simulink model "Full"  (R2014b)
settings: Solver=ode45  StartTime=5  StopTime=Timemax  RelTol=1e-3
values from neighbouring files (symbols this model uses):
  params = fillPosEstimatorInavParams(Par)    [a_log_read.m]
  SampleTime = ts    [a_log_read.m]
undefined symbols (not defined in the file or in its folder): Par, ts
libraries: mylib x10, dspsigattribs x1
settings Model: Creator=Marat  LastModifiedBy=Marat

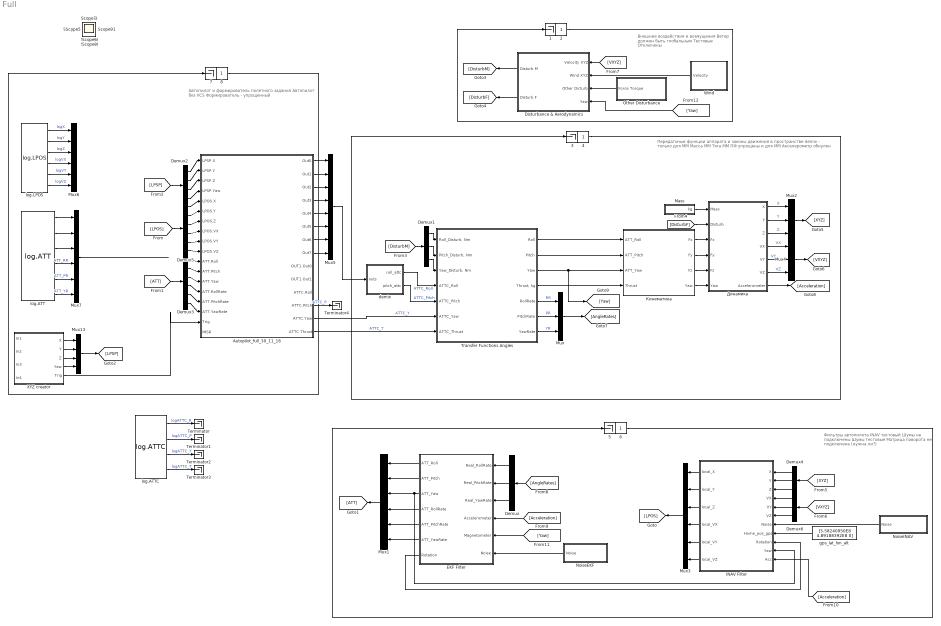
== system Full ==
  note: Передатоные функции аппарата и законы движения в пространстве
      | demix - только для ММ
      | Масса ММ
      | Тяга ММ
      | ПФ упрощены и для ММ
      | Акселерометр обнулен
  note: Внешние воздействия и возмущения
      | Ветер должен быть глобальным
      | Тестовые
      | Отключены
  note: Фильтры автопилота
      | INAV тестовый
      | Шумы не подключены
      | Шумы тестовые
      | Матрица поворота не подключена (нужна ли?)
  note: Автопилот и формирователь полетного задания
      | Автопилот без VCS
      | Формирователь - упрощенный
  {1,3,5,7} (4 alike) : Terminator
  {2,4,6,8} (4 alike) : Constant
  Autopilot_full_30_11_16 : Subsystem  AncestorBlock=mylib/Autopilot_full_30_11_16  mask(Автопилот полный pos + attitude){}
      mask help:
      | Автопилот полный 30.11.16 для анализа в полном автомате
      | (полет по GPS)
      mask Help:
      | Автор - М.Сабиров
      | 30.11.16
  Demux{,1,4,6} (4 alike) : Demux  Outputs=3
  Demux2 : Demux
  Demux3 : Demux  Outputs=6
  Demux5 : Demux  Outputs=6
  Disturbance & Aerodynamics : Subsystem
  EKF Filter : Subsystem
  INAV Filter : Subsystem
  Mass : Subsystem
  Mux : Mux  Inputs=3
  Mux{1,3,6..7} (4 alike) : Mux  Inputs=6
  Mux13 : Mux
  Mux2 : Mux  Inputs=3
  Mux4 : Mux  Inputs=3
  Mux5 : Mux  Inputs=8
  NoiseEKF : Subsystem
  NoiseINAV : Subsystem
  Other Disturbance : Subsystem
  Terminator{,1..4} (5 alike) : Terminator
  Transfer Functions Angles : Subsystem
  Wind : Subsystem
  XYZ creator : Subsystem
  demix : Subsystem
  gps_lat_lon_alt : Constant  Value=[5.58240950E8 4.89188392E8 0]
  log.ATT : mylib/Log_read/log.ATT
  log.ATTC : mylib/Log_read/log.ATTC
  log.LPOS : mylib/Log_read/log.LPOS
  Динамика : Subsystem
  Кинематика : MATLAB Function  TreatAsAtomicUnit=on
  Scope{,1..13} (14 alike) : Scope
      Scope settings: ShowLegends=on  YMin=-2.5  YMax=2.5
      Scope1 settings: ShowLegends=on  YMin=-2  YMax=1
      Scope10 settings: ShowLegends=on  YMin=-0.5  YMax=0.4  SaveName=ScopeData14
      Scope11 settings: ShowLegends=on  YMin=-0.3  YMax=0.4  SaveName=ScopeData17
      Scope12 settings: ShowLegends=on  YMin=-6  YMax=8  SaveName=ScopeData19
      Scope13 settings: ShowLegends=on  SaveName=ScopeData20
      Scope2 settings: ShowLegends=on  YMin=-0.5  YMax=0.2  SaveName=ScopeData2
      Scope3 settings: SaveName=ScopeData3
      Scope4 settings: ShowLegends=on  YMin=-2.5  YMax=0.5  SaveName=ScopeData4
      Scope5 settings: ShowLegends=on  YMin=0.65  YMax=0.95  SaveName=ScopeData6
      Scope6 settings: ShowLegends=on  SaveName=ScopeData18
      Scope7 settings: ShowLegends=on  YMin=-12  YMax=0  SaveName=ScopeData8
      Scope8 settings: ShowLegends=on  TimeRange=19.50883891213388  YMin=-0.18  YMax=-0.04  SaveName=ScopeData11
      Scope9 settings: ShowLegends=on  TimeRange=102.475  YMin=-30  YMax=15  SaveName=ScopeData12
  wires:
  Autopilot_full_30_11_16/13(ATTC.Yaw) -> Transfer Functions Angles/6(ATTC_Yaw)  "ATTC_Y"
  Autopilot_full_30_11_16/14(ATTC.Thrust) -> Transfer Functions Angles/7(ATTC_Thrust)  "ATTC_T"
  Transfer Functions Angles/7(YawRate) -> Mux/3  "YR"
  Transfer Functions Angles/6(PitchRate) -> Mux/2  "PR"
  Transfer Functions Angles/5(RollRate) -> Mux/1  "RR"
  Demux/1 -> EKF Filter/1(Real_RollRate)
  Demux/2 -> EKF Filter/2(Real_PitchRate)
  Demux/3 -> EKF Filter/3(Real_YawRate)
  Demux1/3 -> Transfer Functions Angles/3("Yaw_Disturb, Nm")
  Demux1/2 -> Transfer Functions Angles/2("Pitch_Disturb, Nm")
  Demux1/1 -> Transfer Functions Angles/1("Roll_Disturb, Nm")
  EKF Filter/1(ATT_Roll) -> Mux1/1
  EKF Filter/6(ATT_YawRate) -> Mux1/6
  Demux3/1 -> Autopilot_full_30_11_16/11(ATT.Roll)
  Demux3/6 -> Autopilot_full_30_11_16/16(ATT.YawRate)
  Demux3/5 -> Autopilot_full_30_11_16/15(ATT.PitchRate)
  Demux3/4 -> Autopilot_full_30_11_16/14(ATT.RollRate)
  Demux3/3 -> Autopilot_full_30_11_16/13(ATT.Yaw)
  Demux3/2 -> Autopilot_full_30_11_16/12(ATT.Pitch)
  EKF Filter/2(ATT_Pitch) -> Mux1/2
  EKF Filter/3(ATT_Yaw) -> INAV Filter/10(Yaw), Mux1/3
  EKF Filter/4(ATT_RollRate) -> Mux1/4
  EKF Filter/5(ATT_PitchRate) -> Mux1/5
  Transfer Functions Angles/1(Roll) -> Кинематика/1(ATT_Roll)
  Transfer Functions Angles/2(Pitch) -> Кинематика/2(ATT_Pitch)
  Transfer Functions Angles/3(Yaw) -> Кинематика/3(ATT_Yaw), [Yaw]
  Кинематика/1(Fx) -> Динамика/3(Fx)
  Кинематика/2(Fy) -> Динамика/4(Fy)
  Динамика/1(X) -> Mux2/1  "X"
  Динамика/2(Y) -> Mux2/2  "Y"
  Динамика/3(Z) -> Mux2/3  "Z"
  Динамика/4(VX) -> Mux4/1  "VX"
  Динамика/5(VY) -> Mux4/2  "VY"
  Динамика/6(VZ) -> Mux4/3  "VZ"
  Demux4/1 -> INAV Filter/1(X)
  Demux6/3 -> INAV Filter/6(VZ)
  Demux6/2 -> INAV Filter/5(VY)
  Demux6/1 -> INAV Filter/4(VX)
  Demux4/3 -> INAV Filter/3(Z)
  INAV Filter/1(local_X) -> Mux3/1
  INAV Filter/6(local_VZ) -> Mux3/6
  INAV Filter/2(local_Y) -> Mux3/2
  INAV Filter/3(local_Z) -> Mux3/3
  INAV Filter/4(local_VX) -> Mux3/4
  INAV Filter/5(local_VY) -> Mux3/5
  Demux4/2 -> INAV Filter/2(Y)
  Demux5/1 -> Autopilot_full_30_11_16/5(LPOS.X)
  Demux5/6 -> Autopilot_full_30_11_16/10(LPOS.VZ)
  Demux5/5 -> Autopilot_full_30_11_16/9(LPOS.VY)
  Demux5/4 -> Autopilot_full_30_11_16/8(LPOS.VX)
  Demux5/3 -> Autopilot_full_30_11_16/7(LPOS.Z)
  Demux5/2 -> Autopilot_full_30_11_16/6(LPOS.Y)
  Other Disturbance/1(Force Torque) -> Disturbance & Aerodynamics/3(Other Dicturb)
  NoiseINAV/1(Noise) -> INAV Filter/7(Noise)
  NoiseEKF/1(Noise) -> EKF Filter/6(Noise)
  EKF Filter/7(Rotation) -> INAV Filter/9(Rotation)
  gps_lat_lon_alt/1 -> INAV Filter/8(Home_pos_gps)
  XYZ creator/5(Trig) -> Autopilot_full_30_11_16/17(Trig)
  log.LPOS/1 -> Mux6/1  "logX"
  log.LPOS/6 -> Mux6/6  "logVZ"
  log.LPOS/2 -> Mux6/2  "logY"
  log.LPOS/3 -> Mux6/3  "logZ"
  log.LPOS/4 -> Mux6/4  "logVX"
  log.LPOS/5 -> Mux6/5  "logVY"
  log.ATT/1 -> Mux7/1
  log.ATT/2 -> Mux7/2
  log.ATT/3 -> Mux7/3
  log.ATT/4 -> Mux7/4  "ATT_RR"
  log.ATT/5 -> Mux7/5  "ATT_PR"
  log.ATT/6 -> Mux7/6  "ATT_YR"
  [LPOS] -> Demux5/1
  Mux3/1 -> [LPOS]
  Mux7/1 -> ?
  Mux1/1 -> [ATT]
  XYZ creator/1(X) -> Mux13/1
  XYZ creator/2(Y) -> Mux13/2
  XYZ creator/3(Z) -> Mux13/3
  XYZ creator/4(Yaw) -> Mux13/4
  Demux2/4 -> Autopilot_full_30_11_16/4(LPSP.Yaw)
  Demux2/1 -> Autopilot_full_30_11_16/1(LPSP.X)
  Demux2/2 -> Autopilot_full_30_11_16/2(LPSP.Y)
  Demux2/3 -> Autopilot_full_30_11_16/3(LPSP.Z)
  Mux13/1 -> [LPSP]
  [LPSP] -> Demux2/1
  [DisturbM] -> Demux1/1
  Disturbance & Aerodynamics/1(Disturb M) -> [DisturbM]
  Disturbance & Aerodynamics/2(Disturb F) -> [DisturbF]
  [DisturbF] -> Динамика/2(Disturb)
  Mux2/1 -> [XYZ]
  [XYZ] -> Demux4/1
  Mux4/1 -> [VXYZ]
  [VXYZ] -> Demux6/1
  [VXYZ] -> Disturbance & Aerodynamics/1(Velocity XYZ)
  Mux/1 -> [AngleRates]
  [AngleRates] -> Demux/1
  Динамика/7(Accelerometer) -> [Acceleration]
  [Acceleration] -> EKF Filter/4(Accelerometer)
  [Acceleration] -> INAV Filter/11(Acc)
  [Yaw] -> EKF Filter/5(Magnetometer)
  4/1 -> 3/1
  6/1 -> 5/1
  2/1 -> 1/1
  8/1 -> 7/1
  log.ATTC/1 -> Terminator/1  "logATTC_R"
  log.ATTC/2 -> Terminator1/1  "logATTC_P"
  log.ATTC/3 -> Terminator2/1  "logATTC_Y"
  log.ATTC/4 -> Terminator3/1  "logATTC_T"
  demix/2(pitch_attc) -> Transfer Functions Angles/5(ATTC_Pitch)  "ATTC_Pitch"
  Autopilot_full_30_11_16/1(Out0) -> Mux5/1
  Autopilot_full_30_11_16/8(Out7) -> Mux5/8
  Autopilot_full_30_11_16/2(Out1) -> Mux5/2
  Autopilot_full_30_11_16/3(Out2) -> Mux5/3
  Autopilot_full_30_11_16/5(Out4) -> Mux5/5
  Autopilot_full_30_11_16/7(Out6) -> Mux5/7
  Autopilot_full_30_11_16/6(Out5) -> Mux5/6
  Autopilot_full_30_11_16/4(Out3) -> Mux5/4
  Mux5/1 -> demix/1(outs)
  demix/1(roll_attc) -> Transfer Functions Angles/4(ATTC_Roll)  "ATTC_Roll"
  Mass/1(kg) -> Динамика/1(Mass)
  [Yaw] -> Disturbance & Aerodynamics/4(Yaw)
  Wind/1(Velocity) -> Disturbance & Aerodynamics/2(Wind XYZ)
  Autopilot_full_30_11_16/12(ATTC.Pitch) -> Terminator4/1  "ATTC_P"
  [ATT] -> Demux3/1
  Transfer Functions Angles/4("Thrust, kg") -> Кинематика/4(Thrust)
  Кинематика/3(Fz) -> Динамика/5(Fz)
  Кинематика/4(Yaw) -> Динамика/6(Yaw)

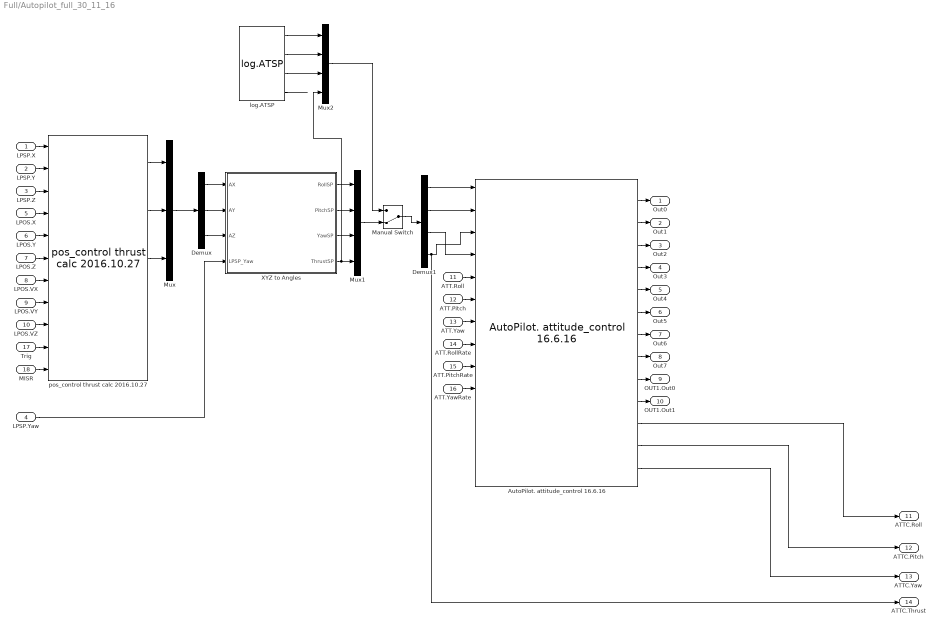
== system Full/Autopilot_full_30_11_16 ==
  LPSP.X : Inport
  LPSP.Y : Inport  Port=2
  LPSP.Z : Inport  Port=3
  LPSP.Yaw : Inport  Port=4
  LPOS.X : Inport  Port=5
  LPOS.Y : Inport  Port=6
  LPOS.Z : Inport  Port=7
  LPOS.VX : Inport  Port=8
  LPOS.VY : Inport  Port=9
  LPOS.VZ : Inport  Port=10
  ATT.Roll : Inport  Port=11
  ATT.Pitch : Inport  Port=12
  ATT.Yaw : Inport  Port=13
  ATT.RollRate : Inport  Port=14
  ATT.PitchRate : Inport  Port=15
  ATT.YawRate : Inport  Port=16
  Trig : Inport  Port=17
  MISR : Inport  Port=18
  AutoPilot. attitude_control 16.6.16 : mylib/AutoPilot. attitude_control  16.6.16  log_model=off  mm_model=off  rotation_yaw=on
  Demux : Demux  Outputs=3
  Demux1 : Demux
  Manual Switch : ManualSwitch  CurrentSetting=0
  Mux : Mux  Inputs=3
  Mux1 : Mux
  Mux2 : Mux
  XYZ to Angles : MATLAB Function  TreatAsAtomicUnit=on  mask(Преобразование желаемого вектора тяги в углы управления){}
      mask help:
      | Входами блока являются выходы Pos_Control:
      |     AX - проекция желаемой тяги на Х
      |     AY - проекция желаемой тяги на Y
      |     AZ - проекция желаемой тяги на Z
      | и желаемое рыскание LPSP.Yaw
      |
      | Выходами блока являются входы Att_Control:
      |     RollSP - желаемый угол наклона по крену,
      |     PitchSP - желаемый угол наклона по тангажу,
      |     YawSP  - желаемый угол наклона по рысканию,
      |     ThrustSP - желаемая тяга.
  log.ATSP : mylib/Log_read/log.ATSP
  pos_control thrust calc 2016.10.27 : mylib/pos_control thrust calc 2016.10.27
  Out0 : Outport
  Out1 : Outport  Port=2
  Out2 : Outport  Port=3
  Out3 : Outport  Port=4
  Out4 : Outport  Port=5
  Out5 : Outport  Port=6
  Out6 : Outport  Port=7
  Out7 : Outport  Port=8
  OUT1.Out0 : Outport  Port=9
  OUT1.Out1 : Outport  Port=10
  ATTC.Roll : Outport  Port=11
  ATTC.Pitch : Outport  Port=12
  ATTC.Yaw : Outport  Port=13
  ATTC.Thrust : Outport  Port=14
  wires:
  AutoPilot. attitude_control 16.6.16/10 -> OUT1.Out1/1
  AutoPilot. attitude_control 16.6.16/9 -> OUT1.Out0/1
  pos_control thrust calc 2016.10.27/1 -> Mux/1
  pos_control thrust calc 2016.10.27/2 -> Mux/2
  pos_control thrust calc 2016.10.27/3 -> Mux/3
  Mux/1 -> Demux/1
  Demux/1 -> XYZ to Angles/1(AX)
  Demux/2 -> XYZ to Angles/2(AY)
  Demux/3 -> XYZ to Angles/3(AZ)
  XYZ to Angles/1(RollSP) -> Mux1/1
  XYZ to Angles/2(PitchSP) -> Mux1/2
  XYZ to Angles/3(YawSP) -> Mux1/3
  XYZ to Angles/4(ThrustSP) -> Mux2/4, Mux1/4
  Demux1/1 -> AutoPilot. attitude_control 16.6.16/1
  Demux1/2 -> AutoPilot. attitude_control 16.6.16/2
  Demux1/3 -> AutoPilot. attitude_control 16.6.16/4
  Demux1/4 -> ATTC.Thrust/1, AutoPilot. attitude_control 16.6.16/3
  Mux1/1 -> Manual Switch/2
  ATT.Pitch/1 -> AutoPilot. attitude_control 16.6.16/6
  ATT.YawRate/1 -> AutoPilot. attitude_control 16.6.16/10
  ATT.PitchRate/1 -> AutoPilot. attitude_control 16.6.16/9
  ATT.Yaw/1 -> AutoPilot. attitude_control 16.6.16/7
  ATT.RollRate/1 -> AutoPilot. attitude_control 16.6.16/8
  ATT.Roll/1 -> AutoPilot. attitude_control 16.6.16/5
  LPOS.VX/1 -> pos_control thrust calc 2016.10.27/7
  AutoPilot. attitude_control 16.6.16/11 -> ATTC.Roll/1
  LPOS.VZ/1 -> pos_control thrust calc 2016.10.27/9
  AutoPilot. attitude_control 16.6.16/1 -> Out0/1
  LPOS.VY/1 -> pos_control thrust calc 2016.10.27/8
  LPOS.Y/1 -> pos_control thrust calc 2016.10.27/5
  LPOS.X/1 -> pos_control thrust calc 2016.10.27/4
  LPOS.Z/1 -> pos_control thrust calc 2016.10.27/6
  AutoPilot. attitude_control 16.6.16/5 -> Out4/1
  AutoPilot. attitude_control 16.6.16/8 -> Out7/1
  AutoPilot. attitude_control 16.6.16/6 -> Out5/1
  AutoPilot. attitude_control 16.6.16/3 -> Out2/1
  AutoPilot. attitude_control 16.6.16/2 -> Out1/1
  AutoPilot. attitude_control 16.6.16/7 -> Out6/1
  AutoPilot. attitude_control 16.6.16/4 -> Out3/1
  AutoPilot. attitude_control 16.6.16/12 -> ATTC.Pitch/1
  AutoPilot. attitude_control 16.6.16/13 -> ATTC.Yaw/1
  LPSP.Yaw/1 -> XYZ to Angles/4(LPSP_Yaw)
  LPSP.Y/1 -> pos_control thrust calc 2016.10.27/2
  LPSP.Z/1 -> pos_control thrust calc 2016.10.27/3
  LPSP.X/1 -> pos_control thrust calc 2016.10.27/1
  Trig/1 -> pos_control thrust calc 2016.10.27/10
  MISR/1 -> pos_control thrust calc 2016.10.27/11
  log.ATSP/1 -> Mux2/1
  log.ATSP/2 -> Mux2/2
  log.ATSP/3 -> Mux2/3
  log.ATSP/4 -> ?
  Mux2/1 -> Manual Switch/1
  Manual Switch/1 -> Demux1/1

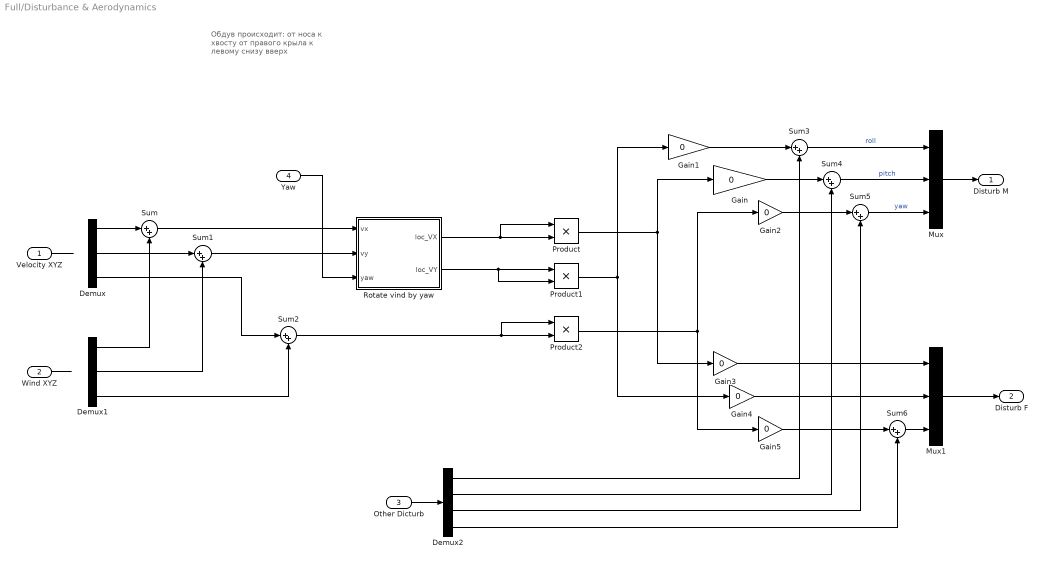
== system Full/Disturbance & Aerodynamics ==
  note: Обдув происходит:
      | от носа к хвосту
      | от правого крыла к левому
      | снизу вверх
  Velocity XYZ : Inport
  Wind XYZ : Inport  Port=2
  Other Dicturb : Inport  Port=3
  Yaw : Inport  Port=4
  Demux : Demux  Outputs=3
  Demux1 : Demux  Outputs=3
  Demux2 : Demux
  Gain{,1..5} (6 alike) : Gain  Gain=0
  Mux : Mux  Inputs=3
  Mux1 : Mux  Inputs=3
  Product : Product
  Product1 : Product
  Product2 : Product
  Rotate vind by yaw : MATLAB Function  TreatAsAtomicUnit=on
  Sum{,1..6} (7 alike) : Sum  Inputs=|++
  Disturb M : Outport
  Disturb F : Outport  Port=2
  wires:
  Mux/1 -> Disturb M/1
  Mux1/1 -> Disturb F/1
  Velocity XYZ/1 -> ?
  Wind XYZ/1 -> ?
  Demux/1 -> Sum/1
  Demux1/1 -> Sum/2
  Demux/2 -> Sum1/1
  Demux1/2 -> Sum1/2
  Demux/3 -> Sum2/1
  Demux1/3 -> Sum2/2
  Sum/1 -> Rotate vind by yaw/1(vx)
  Sum1/1 -> Rotate vind by yaw/2(vy)
  Yaw/1 -> Rotate vind by yaw/3(yaw)
  Rotate vind by yaw/1(loc_VX) -> Product/1, Product/2
  Rotate vind by yaw/2(loc_VY) -> Product1/2, Product1/1
  Sum2/1 -> Product2/1, Product2/2
  Product/1 -> Gain3/1, Gain/1
  Product1/1 -> Gain4/1, Gain1/1
  Product2/1 -> Gain5/1, Gain2/1
  Sum4/1 -> Mux/2  "pitch"
  Sum3/1 -> Mux/1  "roll"
  Sum5/1 -> Mux/3  "yaw"
  Gain3/1 -> Mux1/1
  Gain4/1 -> Mux1/2
  Gain5/1 -> Sum6/1
  Gain2/1 -> Sum5/1
  Gain/1 -> Sum4/1
  Gain1/1 -> Sum3/1
  Other Dicturb/1 -> Demux2/1
  Demux2/1 -> Sum3/2
  Demux2/2 -> Sum4/2
  Demux2/3 -> Sum5/2
  Sum6/1 -> Mux1/3
  Demux2/4 -> Sum6/2

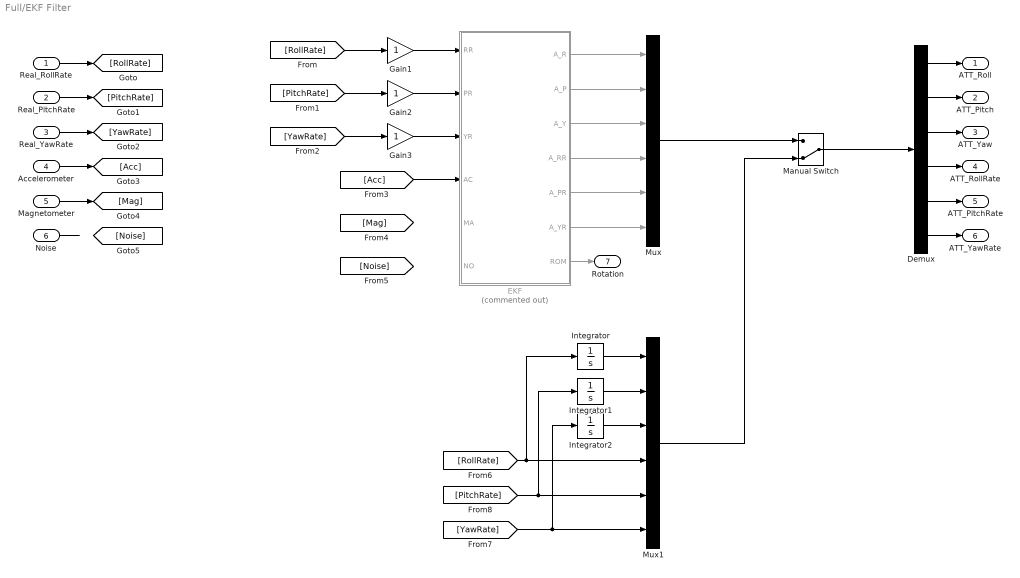
== system Full/EKF Filter ==
  Real_RollRate : Inport
  Real_PitchRate : Inport  Port=2
  Real_YawRate : Inport  Port=3
  Accelerometer : Inport  Port=4
  Magnetometer : Inport  Port=5
  Noise : Inport  Port=6
  Demux : Demux  Outputs=6
  EKF : Subsystem  Commented=on
  Gain1 : Gain  SampleTime=ts
  Gain2 : Gain  SampleTime=ts
  Gain3 : Gain  SampleTime=ts
  Integrator : Integrator
  Integrator1 : Integrator
  Integrator2 : Integrator
  Manual Switch : ManualSwitch  CurrentSetting=0
  Mux : Mux  Inputs=6
  Mux1 : Mux  Inputs=6
  ATT_Roll : Outport
  ATT_Pitch : Outport  Port=2
  ATT_Yaw : Outport  Port=3
  ATT_RollRate : Outport  Port=4
  ATT_PitchRate : Outport  Port=5
  ATT_YawRate : Outport  Port=6
  Rotation : Outport  Port=7
  wires:
  Real_RollRate/1 -> [RollRate]
  Real_PitchRate/1 -> [PitchRate]
  Real_YawRate/1 -> [YawRate]
  Accelerometer/1 -> [Acc]
  Magnetometer/1 -> [Mag]
  Noise/1 -> ?
  [RollRate] -> Gain1/1
  [PitchRate] -> Gain2/1
  [YawRate] -> Gain3/1
  EKF/1(A_R) -> Mux/1
  EKF/7(ROM) -> Rotation/1
  EKF/2(A_P) -> Mux/2
  EKF/3(A_Y) -> Mux/3
  EKF/4(A_RR) -> Mux/4
  EKF/5(A_PR) -> Mux/5
  EKF/6(A_YR) -> Mux/6
  [YawRate] -> Integrator2/1, Mux1/6
  [PitchRate] -> Integrator1/1, Mux1/5
  Integrator/1 -> Mux1/1
  [RollRate] -> Integrator/1, Mux1/4
  Integrator1/1 -> Mux1/2
  Integrator2/1 -> Mux1/3
  Demux/1 -> ATT_Roll/1
  Demux/6 -> ATT_YawRate/1
  Demux/2 -> ATT_Pitch/1
  Demux/3 -> ATT_Yaw/1
  Demux/4 -> ATT_RollRate/1
  Demux/5 -> ATT_PitchRate/1
  Mux/1 -> Manual Switch/1
  Mux1/1 -> Manual Switch/2
  Manual Switch/1 -> Demux/1
  Gain1/1 -> EKF/1(RR)
  Gain2/1 -> EKF/2(PR)
  Gain3/1 -> EKF/3(YR)
  [Acc] -> EKF/4(AC)

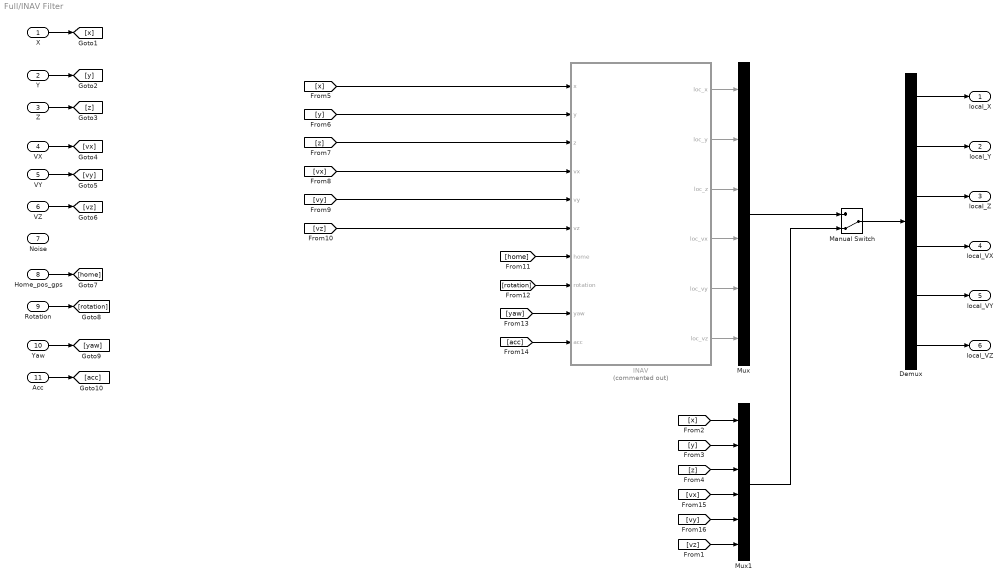
== system Full/INAV Filter ==
  X : Inport
  Y : Inport  Port=2
  Z : Inport  Port=3
  VX : Inport  Port=4
  VY : Inport  Port=5
  VZ : Inport  Port=6
  Noise : Inport  Port=7
  Home_pos_gps : Inport  Port=8
  Rotation : Inport  Port=9
  Yaw : Inport  Port=10
  Acc : Inport  Port=11
  Demux : Demux  Outputs=6
  INAV : Subsystem  Commented=on
  Manual Switch : ManualSwitch  CurrentSetting=0
  Mux : Mux  Inputs=6
  Mux1 : Mux  Inputs=6
  local_X : Outport
  local_Y : Outport  Port=2
  local_Z : Outport  Port=3
  local_VX : Outport  Port=4
  local_VY : Outport  Port=5
  local_VZ : Outport  Port=6
  wires:
  Z/1 -> [z]
  X/1 -> [x]
  Rotation/1 -> [rotation]
  Y/1 -> [y]
  VX/1 -> [vx]
  VY/1 -> [vy]
  VZ/1 -> [vz]
  Home_pos_gps/1 -> [home]
  [rotation] -> INAV/8(rotation)
  Yaw/1 -> [yaw]
  Acc/1 -> [acc]
  [x] -> INAV/1(x)
  [y] -> INAV/2(y)
  [z] -> INAV/3(z)
  [vx] -> INAV/4(vx)
  [vy] -> INAV/5(vy)
  [vz] -> INAV/6(vz)
  [home] -> INAV/7(home)
  [yaw] -> INAV/9(yaw)
  INAV/1(loc_x) -> Mux/1
  INAV/6(loc_vz) -> Mux/6
  INAV/2(loc_y) -> Mux/2
  INAV/3(loc_z) -> Mux/3
  INAV/4(loc_vx) -> Mux/4
  INAV/5(loc_vy) -> Mux/5
  [x] -> Mux1/1
  [y] -> Mux1/2
  [z] -> Mux1/3
  [vx] -> Mux1/4
  [vy] -> Mux1/5
  [vz] -> Mux1/6
  Mux/1 -> Manual Switch/1
  Mux1/1 -> Manual Switch/2
  Manual Switch/1 -> Demux/1
  Demux/1 -> local_X/1
  Demux/2 -> local_Y/1
  Demux/3 -> local_Z/1
  Demux/4 -> local_VX/1
  Demux/5 -> local_VY/1
  Demux/6 -> local_VZ/1
  [acc] -> INAV/10(acc)

== system Full/Mass ==
  Constant : Constant  Value=5.8
  kg : Outport
  wires:
  Constant/1 -> kg/1

== system Full/NoiseEKF ==
  Mux : Mux  Inputs=9
  Sine Wave{,1..8} (9 alike) : Sin  SampleTime=0
  Noise : Outport
  wires:
  Sine Wave/1 -> Mux/1
  Mux/1 -> Noise/1
  Sine Wave1/1 -> Mux/2
  Sine Wave2/1 -> Mux/3
  Sine Wave3/1 -> Mux/4
  Sine Wave4/1 -> Mux/5
  Sine Wave5/1 -> Mux/6
  Sine Wave6/1 -> Mux/7
  Sine Wave7/1 -> Mux/8
  Sine Wave8/1 -> Mux/9

== system Full/NoiseINAV ==
  Mux : Mux  Inputs=3
  Sine Wave : Sin  SampleTime=0
  Sine Wave1 : Sin  SampleTime=0
  Sine Wave2 : Sin  SampleTime=0
  Noise : Outport
  wires:
  Sine Wave2/1 -> Mux/3
  Sine Wave1/1 -> Mux/2
  Mux/1 -> Noise/1
  Sine Wave/1 -> Mux/1

== system Full/Other Disturbance ==
  Constant{,1..3} (4 alike) : Constant
  Mux : Mux
  Force Torque : Outport
  wires:
  Mux/1 -> ?
  Constant/1 -> Mux/1
  Constant1/1 -> Mux/2
  Constant2/1 -> Mux/3
  Constant3/1 -> Mux/4

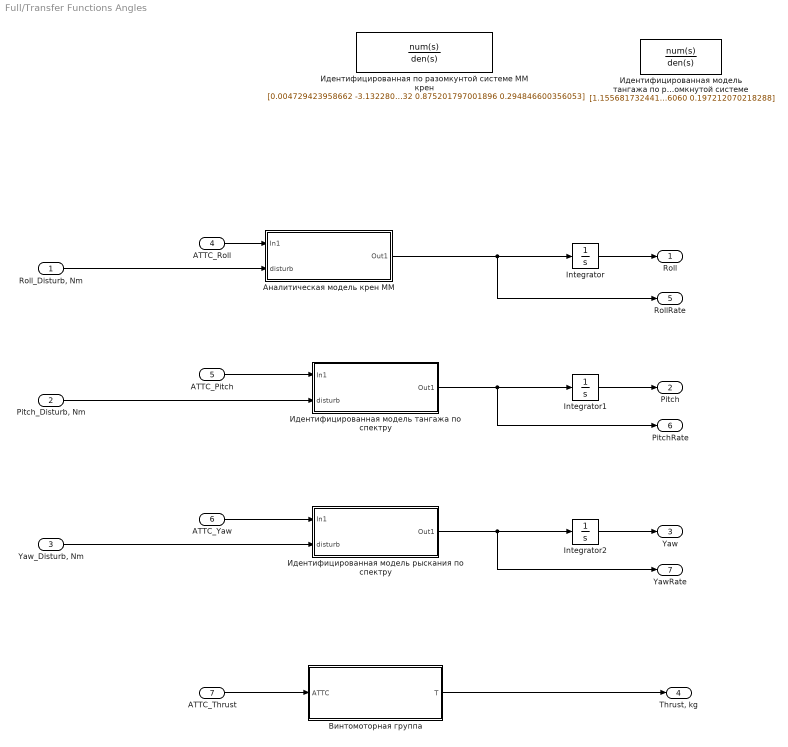
== system Full/Transfer Functions Angles ==
  "Roll_Disturb, Nm" : Inport
  "Pitch_Disturb, Nm" : Inport  Port=2
  "Yaw_Disturb, Nm" : Inport  Port=3
  ATTC_Roll : Inport  Port=4
  ATTC_Pitch : Inport  Port=5
  ATTC_Yaw : Inport  Port=6
  ATTC_Thrust : Inport  Port=7
  Integrator : Integrator
  Integrator1 : Integrator
  Integrator2 : Integrator
  Аналитическая модель крен ММ : Subsystem
  Винтомоторная группа : Subsystem
  Идентифицированная по разомкунтой системе ММ крен : TransferFcn  Numerator=[0.004729423958662 -3.132280434907999 94.756096397393950 1.303168167766560 1.245260396615329e+02 0.115735406235224 13.349760943769445 -0.478364346524675]  Denominator=[1 15.535357249217140 11.955671817027460 26.783502579736705 11.815660799479959 11.550625458961932 0.875201797001896 0.294846600356053]
  Идентифицированная модель рыскания по спектру : Subsystem
  Идентифицированная модель тангажа по разомкнутой системе : TransferFcn  Numerator=[1.155681732441771e+02 -1.453881592237685]  Denominator=[1 7.223948965293692 18.365751375476060 0.197212070218288]
  Идентифицированная модель тангажа по спектру : Subsystem
  Roll : Outport
  Pitch : Outport  Port=2
  Yaw : Outport  Port=3
  "Thrust, kg" : Outport  Port=4
  RollRate : Outport  Port=5
  PitchRate : Outport  Port=6
  YawRate : Outport  Port=7
  wires:
  ATTC_Roll/1 -> Аналитическая модель крен ММ/1(In1)
  ATTC_Pitch/1 -> Идентифицированная модель тангажа по спектру/1(In1)
  ATTC_Yaw/1 -> Идентифицированная модель рыскания по спектру/1(In1)
  ATTC_Thrust/1 -> Винтомоторная группа/1(ATTC)
  Integrator/1 -> Roll/1
  Integrator1/1 -> Pitch/1
  Integrator2/1 -> Yaw/1
  Идентифицированная модель тангажа по спектру/1(Out1) -> PitchRate/1, Integrator1/1
  Идентифицированная модель рыскания по спектру/1(Out1) -> YawRate/1, Integrator2/1
  "Roll_Disturb, Nm"/1 -> Аналитическая модель крен ММ/2(disturb)
  "Pitch_Disturb, Nm"/1 -> Идентифицированная модель тангажа по спектру/2(disturb)
  "Yaw_Disturb, Nm"/1 -> Идентифицированная модель рыскания по спектру/2(disturb)
  Аналитическая модель крен ММ/1(Out1) -> Integrator/1, RollRate/1
  Винтомоторная группа/1(T) -> "Thrust, kg"/1

== system Full/Wind ==
  Mux : Mux  Inputs=3
  Wind velocity from Earth to Sky : Constant  Value=0
  Wind velocity from East to West : Constant  Value=0
  Wind velocity from North no South : Constant  Value=0
  Velocity : Outport
  wires:
  Mux/1 -> Velocity/1
  Wind velocity from North no South/1 -> Mux/1
  Wind velocity from East to West/1 -> Mux/2
  Wind velocity from Earth to Sky/1 -> Mux/3

== system Full/XYZ creator ==
  In1 : Inport
  In2 : Inport  Port=2
  In3 : Inport  Port=3
  In4 : Inport  Port=4
  Constant : Constant  Value=5
  Constant1 : Constant  Value=5
  Constant2 : Constant  Value=5
  Constant4 : Constant  Value=3
  log.LPSP : mylib/Log_read/log.LPSP
  X : Outport
  Y : Outport  Port=2
  Z : Outport  Port=3
  Yaw : Outport  Port=4
  Trig : Outport  Port=5
  wires:
  log.LPSP/1 -> X/1
  log.LPSP/2 -> Y/1
  log.LPSP/3 -> Z/1
  log.LPSP/11 -> Yaw/1
  Constant4/1 -> Trig/1

== system Full/demix ==
  outs : Inport
  Demux : Demux  Outputs=8
  Gain : Gain  Gain=0.5
  Gain1 : Gain  Gain=0.5
  Sum : Sum  Inputs=|+-+-
  Sum1 : Sum  Inputs=|++--
  roll_attc : Outport
  pitch_attc : Outport  Port=2
  wires:
  Demux/1 -> Sum1/1, Sum/1
  Demux/2 -> Sum/2, Sum1/2
  Demux/4 -> Sum/4, Sum1/4
  Demux/3 -> Sum/3, Sum1/3
  Sum1/1 -> Gain1/1
  Sum/1 -> Gain/1
  Gain/1 -> roll_attc/1
  Gain1/1 -> pitch_attc/1
  outs/1 -> Demux/1

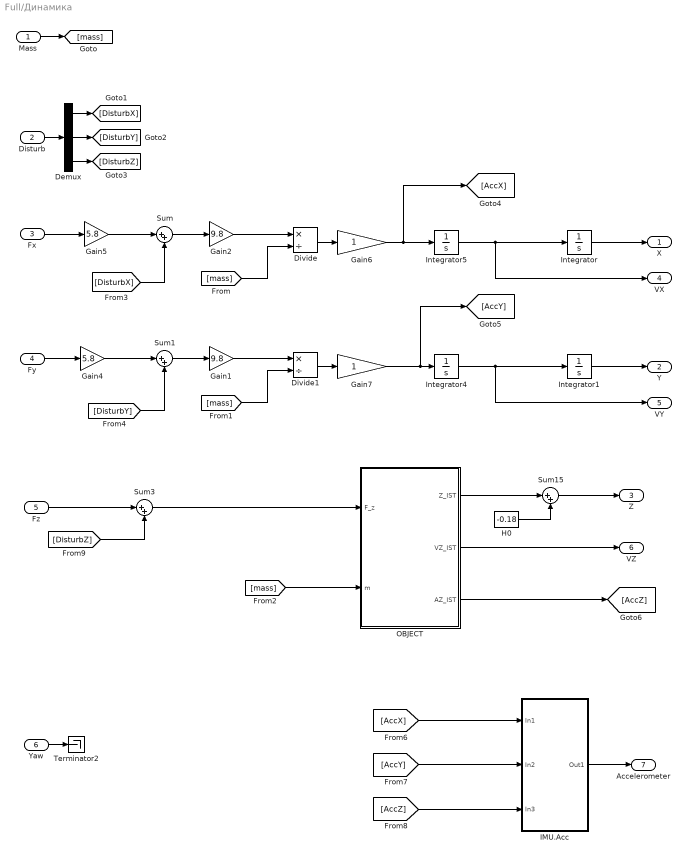
== system Full/Динамика ==
  Mass : Inport
  Disturb : Inport  Port=2
  Fx : Inport  Port=3
  Fy : Inport  Port=4
  Fz : Inport  Port=5
  Yaw : Inport  Port=6
  Demux : Demux  Outputs=3
  Divide : Product  Inputs=*/
  Divide1 : Product  Inputs=*/
  Gain1 : Gain  Gain=9.8
  Gain2 : Gain  Gain=9.8
  Gain4 : Gain  Gain=5.8
  Gain5 : Gain  Gain=5.8
  Gain6 : Gain
  Gain7 : Gain
  H0 : Constant  Value=-0.18
  IMU.Acc : Subsystem
  Integrator : Integrator  InitialCondition=4
  Integrator1 : Integrator  InitialCondition=5
  Integrator4 : Integrator
  Integrator5 : Integrator
  OBJECT : Subsystem
  Sum{,1,3,15} (4 alike) : Sum  Inputs=|++
  Terminator2 : Terminator
  X : Outport
  Y : Outport  Port=2
  Z : Outport  Port=3
  VX : Outport  Port=4
  VY : Outport  Port=5
  VZ : Outport  Port=6
  Accelerometer : Outport  Port=7
  wires:
  Integrator1/1 -> Y/1
  Integrator/1 -> X/1
  Divide1/1 -> Gain7/1
  Divide/1 -> Gain6/1
  Mass/1 -> [mass]
  [mass] -> Divide/2
  [mass] -> Divide1/2
  Gain1/1 -> Divide1/1
  Gain2/1 -> Divide/1
  Integrator4/1 -> VY/1, Integrator1/1
  Integrator5/1 -> Integrator/1, VX/1
  [mass] -> OBJECT/2(m)
  Sum/1 -> Gain2/1
  Sum1/1 -> Gain1/1
  Disturb/1 -> Demux/1
  Fx/1 -> Gain5/1
  Fy/1 -> Gain4/1
  Demux/1 -> [DisturbX]
  Demux/2 -> [DisturbY]
  Demux/3 -> [DisturbZ]
  [DisturbX] -> Sum/2
  [DisturbY] -> Sum1/2
  [AccX] -> IMU.Acc/1(In1)
  [AccY] -> IMU.Acc/2(In2)
  [AccZ] -> IMU.Acc/3(In3)
  IMU.Acc/1(Out1) -> Accelerometer/1
  Gain6/1 -> [AccX], Integrator5/1
  Gain7/1 -> [AccY], Integrator4/1
  Fz/1 -> Sum3/1
  OBJECT/3(AZ_IST) -> [AccZ]
  OBJECT/2(VZ_IST) -> VZ/1
  OBJECT/1(Z_IST) -> Sum15/1
  Sum15/1 -> Z/1
  [DisturbZ] -> Sum3/2
  H0/1 -> Sum15/2
  Gain4/1 -> Sum1/1
  Gain5/1 -> Sum/1
  Sum3/1 -> OBJECT/1(F_z)
  Yaw/1 -> Terminator2/1

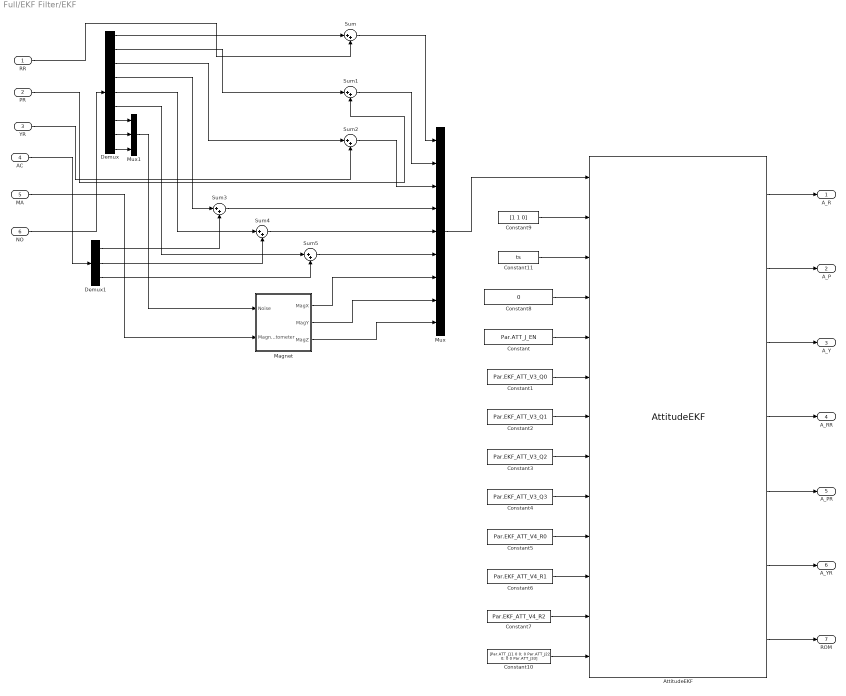
== system Full/EKF Filter/EKF ==
  RR : Inport
  PR : Inport  Port=2
  YR : Inport  Port=3
  AC : Inport  Port=4
  MA : Inport  Port=5
  NO : Inport  Port=6
  AttitudeEKF : mylib/AttitudeEKF
  Constant : Constant  Value=Par.ATT_J_EN
  Constant1 : Constant  Value=Par.EKF_ATT_V3_Q0
  Constant10 : Constant  Value=[Par.ATT_J11 0 0; 0 Par.ATT_J22 0; 0 0 Par.ATT_J33]
  Constant11 : Constant  Value=ts
  Constant2 : Constant  Value=Par.EKF_ATT_V3_Q1
  Constant3 : Constant  Value=Par.EKF_ATT_V3_Q2
  Constant4 : Constant  Value=Par.EKF_ATT_V3_Q3
  Constant5 : Constant  Value=Par.EKF_ATT_V4_R0
  Constant6 : Constant  Value=Par.EKF_ATT_V4_R1
  Constant7 : Constant  Value=Par.EKF_ATT_V4_R2
  Constant8 : Constant  Value=0
  Constant9 : Constant  Value=[1 1 0]
  Demux : Demux  Outputs=9
  Demux1 : Demux  Outputs=3
  Magnet : Subsystem
  Mux : Mux  Inputs=9
  Mux1 : Mux  Inputs=3
  Sum{,1..5} (6 alike) : Sum  Inputs=|++
  A_R : Outport
  A_P : Outport  Port=2
  A_Y : Outport  Port=3
  A_RR : Outport  Port=4
  A_PR : Outport  Port=5
  A_YR : Outport  Port=6
  ROM : Outport  Port=7
  wires:
  AttitudeEKF/4 -> A_RR/1
  PR/1 -> Sum1/2
  Constant8/1 -> AttitudeEKF/4
  Constant1/1 -> AttitudeEKF/6
  Constant4/1 -> AttitudeEKF/9
  RR/1 -> Sum/2
  AttitudeEKF/3 -> A_Y/1
  AttitudeEKF/1 -> A_R/1
  Constant11/1 -> AttitudeEKF/3
  AttitudeEKF/5 -> A_PR/1
  Constant3/1 -> AttitudeEKF/8
  Mux/1 -> AttitudeEKF/1
  Constant7/1 -> AttitudeEKF/12
  Demux/1 -> Sum/1
  Sum/1 -> Mux/1
  YR/1 -> Sum2/2
  Constant10/1 -> AttitudeEKF/13
  Constant5/1 -> AttitudeEKF/10
  Constant9/1 -> AttitudeEKF/2
  NO/1 -> Demux/1
  Sum1/1 -> Mux/2
  Constant/1 -> AttitudeEKF/5
  Sum2/1 -> Mux/3
  Constant2/1 -> AttitudeEKF/7
  AttitudeEKF/2 -> A_P/1
  AttitudeEKF/6 -> A_YR/1
  Constant6/1 -> AttitudeEKF/11
  Magnet/1(MagX) -> Mux/7
  Demux/9 -> Mux1/3
  Demux/7 -> Mux1/1
  Sum4/1 -> Mux/5
  Sum3/1 -> Mux/4
  Sum5/1 -> Mux/6
  Magnet/2(MagY) -> Mux/8
  Demux1/3 -> Sum5/2
  Demux1/2 -> Sum4/2
  Demux1/1 -> Sum3/2
  Demux/3 -> Sum2/1
  AC/1 -> Demux1/1
  Demux/2 -> Sum1/1
  Demux/4 -> Sum3/1
  Demux/6 -> Sum5/1
  Mux1/1 -> Magnet/1(Noise)
  Demux/5 -> Sum4/1
  Magnet/3(MagZ) -> Mux/9
  MA/1 -> Magnet/2(Magnetometer)
  Demux/8 -> Mux1/2
  AttitudeEKF/7 -> ROM/1

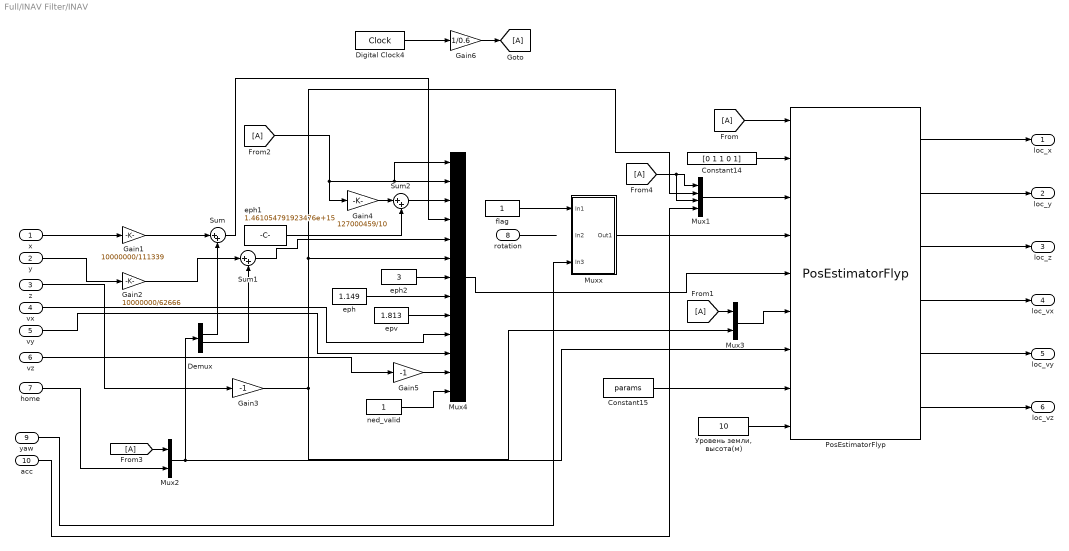
== system Full/INAV Filter/INAV ==
  x : Inport
  y : Inport  Port=2
  z : Inport  Port=3
  vx : Inport  Port=4
  vy : Inport  Port=5
  vz : Inport  Port=6
  home : Inport  Port=7
  rotation : Inport  Port=8
  yaw : Inport  Port=9
  acc : Inport  Port=10
  Constant14 : Constant  Value=[0 1 1 0 1]
  Constant15 : Constant  Value=params  OutDataTypeStr=Bus: slBus1  SampleTime=SampleTime
  Demux : Demux
  Digital Clock4 : DigitalClock  SampleTime=ts
  Gain1 : Gain  Gain=10000000/111339  SampleTime=ts
  Gain2 : Gain  Gain=10000000/62666  SampleTime=ts
  Gain3 : Gain  Gain=-1  SampleTime=ts
  Gain4 : Gain  Gain=127000459/10  SampleTime=ts
  Gain5 : Gain  Gain=-1  SampleTime=ts
  Gain6 : Gain  Gain=1/0.6  SampleTime=ts
  Mux1 : Mux
  Mux2 : Mux  Inputs=2
  Mux3 : Mux  Inputs=2
  Mux4 : Mux  Inputs=13
  Muxx : Subsystem
  PosEstimatorFlyp : mylib/PosEstimatorFlyp
  Sum : Sum  Inputs=|++
  Sum1 : Sum  Inputs=|++
  Sum2 : Sum  Inputs=|++
  eph : Constant  Value=1.149
  eph1 : Constant  Value=1.461054791923476e+15
  eph2 : Constant  Value=3
  epv : Constant  Value=1.813
  flag : Constant
  ned_valid : Constant
  "Уровень земли, высота(м)" : Constant  Value=10  OutDataTypeStr=double  SampleTime=SampleTime
  loc_x : Outport
  loc_y : Outport  Port=2
  loc_z : Outport  Port=3
  loc_vx : Outport  Port=4
  loc_vy : Outport  Port=5
  loc_vz : Outport  Port=6
  wires:
  x/1 -> Gain1/1
  z/1 -> Gain3/1
  rotation/1 -> ?
  Demux/3 -> Sum1/2
  Mux1/1 -> PosEstimatorFlyp/3
  PosEstimatorFlyp/1 -> loc_x/1
  [A] -> PosEstimatorFlyp/1
  eph/1 -> Mux4/8
  vx/1 -> Mux4/10
  ned_valid/1 -> Mux4/13
  y/1 -> Gain2/1
  Mux2/1 -> Demux/1, PosEstimatorFlyp/7
  Constant14/1 -> PosEstimatorFlyp/2
  [A] -> Gain4/1, Mux4/2, Mux4/1
  Gain1/1 -> Sum/1
  Sum/1 -> Mux4/4
  PosEstimatorFlyp/4 -> loc_vx/1
  Mux4/1 -> PosEstimatorFlyp/5
  Demux/2 -> Sum/2
  PosEstimatorFlyp/3 -> loc_z/1
  Constant15/1 -> PosEstimatorFlyp/8
  PosEstimatorFlyp/5 -> loc_vy/1
  PosEstimatorFlyp/6 -> loc_vz/1
  Gain2/1 -> Sum1/1
  vz/1 -> Gain5/1
  PosEstimatorFlyp/2 -> loc_y/1
  epv/1 -> Mux4/9
  "Уровень земли, высота(м)"/1 -> PosEstimatorFlyp/9
  vy/1 -> Mux4/11
  [A] -> Mux2/1
  [A] -> Mux3/1
  home/1 -> Mux2/2
  Gain3/1 -> Mux1/2, Mux4/6, Mux3/2
  Mux3/1 -> PosEstimatorFlyp/6
  flag/1 -> Muxx/1(In1)
  Sum2/1 -> Mux4/3
  yaw/1 -> Muxx/3(In3)
  eph1/1 -> Sum2/2
  Gain4/1 -> Sum2/1
  acc/1 -> Mux1/4
  Muxx/1(Out1) -> PosEstimatorFlyp/4
  Gain5/1 -> Mux4/12
  Sum1/1 -> Mux4/5
  [A] -> Mux1/3, Mux1/1
  eph2/1 -> Mux4/7
  Digital Clock4/1 -> Gain6/1
  Gain6/1 -> [A]

== system Full/Transfer Functions Angles/Аналитическая модель крен ММ ==
  In1 : Inport
  disturb : Inport  Port=2
  Sum : Sum  Inputs=|++
  Инерция и демпф : TransferFcn  Numerator=[1.17]  Denominator=[0.5 1]
  УД ММ : TransferFcn  Numerator=[4.265]  Denominator=[0.22 1]
  Out1 : Outport
  wires:
  Sum/1 -> Инерция и демпф/1
  Инерция и демпф/1 -> Out1/1
  In1/1 -> УД ММ/1
  УД ММ/1 -> Sum/1
  disturb/1 -> Sum/2

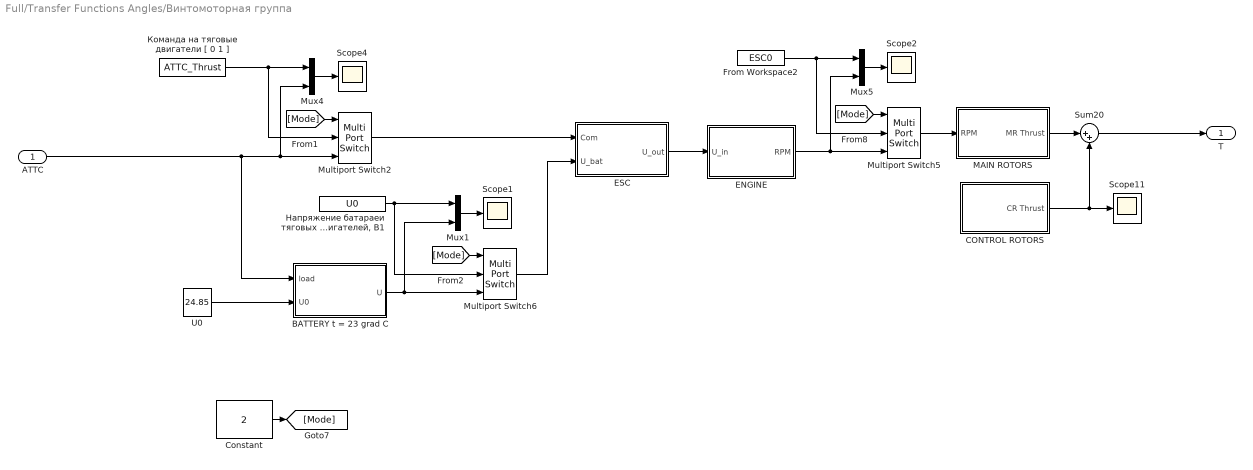
== system Full/Transfer Functions Angles/Винтомоторная группа ==
  ATTC : Inport
  BATTERY t = 23 grad C : Subsystem
  CONTROL ROTORS : Subsystem
  Constant : Constant  Value=2
  ENGINE : Subsystem
  ESC : Subsystem
  From Workspace2 : FromWorkspace  VariableName=ESC0  SampleTime=0.005
  MAIN ROTORS : Subsystem
  Multiport Switch2 : MultiPortSwitch  Inputs=2
  Multiport Switch5 : MultiPortSwitch  Inputs=2
  Multiport Switch6 : MultiPortSwitch  Inputs=2
  Mux1 : Mux  Inputs=2
  Mux4 : Mux  Inputs=2
  Mux5 : Mux  Inputs=2
  Scope{1..2,4,11} (4 alike) : Scope
      Scope1 settings: TimeRange=2  YMin=22.7  YMax=22.9  SaveName=T_com1
      Scope11 settings: TimeRange=2  YMin=0  YMax=1  SaveName=T_com30
      Scope2 settings: TimeRange=2  YMin=7050  YMax=7400  SaveName=T_comgg
      Scope4 settings: TimeRange=102.475  YMin=0.1  YMax=1  SaveName=T_com
  Sum20 : Sum  Inputs=|++
  U0 : Constant  Value=24.85
  Команда на тяговые двигатели [ 0 1 ] : FromWorkspace  VariableName=ATTC_Thrust  SampleTime=ts
  "Напряжение батараеи тяговых двигателей, В1" : FromWorkspace  VariableName=U0  SampleTime=ts
  T : Outport
  wires:
  "Напряжение батараеи тяговых двигателей, В1"/1 -> Multiport Switch6/2, Mux1/1
  Mux5/1 -> Scope2/1
  Multiport Switch5/1 -> MAIN ROTORS/1(RPM)
  From Workspace2/1 -> Multiport Switch5/2, Mux5/1
  [Mode] -> Multiport Switch2/1
  Mux1/1 -> Scope1/1
  BATTERY t = 23 grad C/1(U) -> Multiport Switch6/3, Mux1/2
  ENGINE/1(RPM) -> Mux5/2, Multiport Switch5/3
  CONTROL ROTORS/1(CR Thrust) -> Scope11/1, Sum20/2
  U0/1 -> BATTERY t = 23 grad C/2(U0)
  ESC/1(U_out) -> ENGINE/1(U_in)
  [Mode] -> Multiport Switch6/1
  Команда на тяговые двигатели [ 0 1 ]/1 -> Multiport Switch2/2, Mux4/1
  ATTC/1 -> BATTERY t = 23 grad C/1(load), Mux4/2, Multiport Switch2/3
  [Mode] -> Multiport Switch5/1
  Mux4/1 -> Scope4/1
  Multiport Switch2/1 -> ESC/1(Com)
  MAIN ROTORS/1(MR Thrust) -> Sum20/1
  Constant/1 -> [Mode]
  Sum20/1 -> T/1
  Multiport Switch6/1 -> ESC/2(U_bat)

== system Full/Transfer Functions Angles/Идентифицированная модель рыскания по спектру ==
  In1 : Inport
  disturb : Inport  Port=2
  Gain : Gain
  Sum : Sum  Inputs=|++
  Инерция и демпф1 : TransferFcn  Denominator=[0.7 1]
  УД ММ : TransferFcn  Denominator=[0.25 1]
  Out1 : Outport
  wires:
  In1/1 -> УД ММ/1
  Sum/1 -> Инерция и демпф1/1
  Gain/1 -> Out1/1
  Инерция и демпф1/1 -> Gain/1
  УД ММ/1 -> Sum/1
  disturb/1 -> Sum/2

== system Full/Transfer Functions Angles/Идентифицированная модель тангажа по спектру ==
  In1 : Inport
  disturb : Inport  Port=2
  Gain : Gain  Gain=4
  Sum : Sum  Inputs=|++
  Инерция и демпф : TransferFcn  Denominator=[0.085 1]
  УД ММ : TransferFcn  Numerator=[2.5]  Denominator=[0.22 1]
  Out1 : Outport
  wires:
  Gain/1 -> Out1/1
  Sum/1 -> Инерция и демпф/1
  Инерция и демпф/1 -> Gain/1
  In1/1 -> УД ММ/1
  УД ММ/1 -> Sum/1
  disturb/1 -> Sum/2

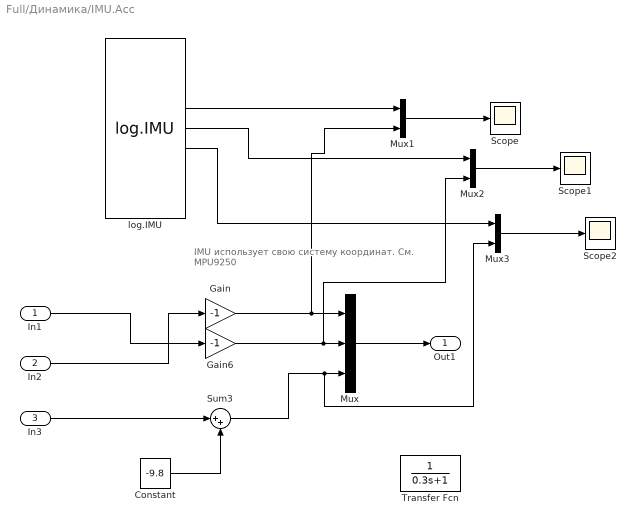
== system Full/Динамика/IMU.Acc ==
  note: IMU использует свою систему координат.
      | См. MPU9250
  In1 : Inport
  In2 : Inport  Port=2
  In3 : Inport  Port=3
  Constant : Constant  Value=-9.8
  Gain : Gain  Gain=-1
  Gain6 : Gain  Gain=-1
  Mux : Mux  Inputs=3
  Mux1 : Mux  Inputs=2
  Mux2 : Mux  Inputs=2
  Mux3 : Mux  Inputs=2
  Scope : Scope
      settings: SaveName=ScopeData23
  Scope1 : Scope
      settings: SaveName=ScopeData24
  Scope2 : Scope
      settings: SaveName=ScopeData25
  Sum3 : Sum  Inputs=|++
  Transfer Fcn : TransferFcn  Denominator=[0.3 1]
  log.IMU : mylib/Log_read/log.IMU
  Out1 : Outport
  wires:
  In1/1 -> Gain6/1
  In2/1 -> Gain/1
  In3/1 -> Sum3/1
  Constant/1 -> Sum3/2
  Mux/1 -> Out1/1
  Gain6/1 -> Mux2/2, Mux/2
  log.IMU/4 -> Mux1/1
  Mux1/1 -> Scope/1
  Mux2/1 -> Scope1/1
  log.IMU/5 -> Mux2/1
  Mux3/1 -> Scope2/1
  log.IMU/6 -> Mux3/1
  Sum3/1 -> Mux3/2, Mux/3
  Gain/1 -> Mux1/2, Mux/1

== system Full/Динамика/OBJECT ==
  F_z : Inport
  m : Inport  Port=2
  AIR RESISTANCE : Subsystem
  DYNAMICS : Subsystem
  GROUND : Subsystem
  GROUND EFFECT : Subsystem
  Memory1 : Memory
  Product3 : Product
  Sum1 : Sum  Inputs=|++
  Z_IST : Outport
  VZ_IST : Outport  Port=2
  AZ_IST : Outport  Port=3
  wires:
  DYNAMICS/1(Az_dyn) -> GROUND/1(Az_dyn)
  m/1 -> DYNAMICS/2(MASS), GROUND/3(MASS)
  DYNAMICS/2(Tz) -> GROUND/2(Tz)
  GROUND/1(Az) -> AZ_IST/1
  AIR RESISTANCE/1(Resistance) -> Sum1/2
  Product3/1 -> Sum1/1, AIR RESISTANCE/1(T)
  Memory1/1 -> GROUND EFFECT/1(H_shassi)
  Sum1/1 -> DYNAMICS/1(T_sum)
  GROUND EFFECT/1(K) -> Product3/2
  GROUND/2(Vz) -> AIR RESISTANCE/2(Vz), VZ_IST/1
  GROUND/3(Z) -> Memory1/1, Z_IST/1
  F_z/1 -> Product3/1

== system Full/EKF Filter/EKF/Magnet ==
  Noise : Inport
  Magnetometer : Inport  Port=2
  Constant : Constant  Value=0
  Constant1 : Constant  Value=0
  Demux : Demux  Outputs=3
  Sum : Sum  Inputs=|++
  Sum1 : Sum  Inputs=|++
  Sum2 : Sum  Inputs=|++
  MagX : Outport
  MagY : Outport  Port=2
  MagZ : Outport  Port=3
  wires:
  Sum1/1 -> MagY/1
  Sum2/1 -> MagZ/1
  Sum/1 -> MagX/1
  Constant/1 -> Sum/2
  Magnetometer/1 -> Sum1/2
  Constant1/1 -> Sum2/2
  Noise/1 -> Demux/1
  Demux/1 -> Sum/1
  Demux/2 -> Sum1/1
  Demux/3 -> Sum2/1

== system Full/INAV Filter/INAV/Muxx ==
  In1 : Inport
  In2 : Inport  Port=2
  In3 : Inport  Port=3
  Convert 2-D to 1-D : dspsigattribs/Convert 2-D to 1-D
  Demux1 : Demux  Outputs=9
  Mux : Mux  Inputs=11
  Out1 : Outport
  wires:
  In1/1 -> Mux/1
  In2/1 -> Convert 2-D to 1-D/1
  Mux/1 -> Out1/1
  Demux1/5 -> Mux/6
  Demux1/9 -> Mux/10
  Demux1/4 -> Mux/5
  In3/1 -> Mux/11
  Demux1/3 -> Mux/4
  Demux1/6 -> Mux/7
  Demux1/1 -> Mux/2
  Demux1/2 -> Mux/3
  Demux1/8 -> Mux/9
  Demux1/7 -> Mux/8
  Convert 2-D to 1-D/1 -> Demux1/1

== system Full/Transfer Functions Angles/Винтомоторная группа/BATTERY t = 23 grad C ==
  load : Inport
  U0 : Inport  Port=2
  Fcn : Fcn  Expr="-2.142 * u(1)^4  -0.8358 * u(1)^3 -1.824 * u(1)^2 -0.09138 * u(1)"
  Gain : Gain  Gain=1/100
  Integrator : Integrator
  Scope4 : Scope
      settings: TimeRange=2  YMin=0.73  YMax=0.82  SaveName=T_com2
  Sum1 : Sum  Inputs=|+-
  Sum3 : Sum  Inputs=|++
  U : Outport
  wires:
  Sum3/1 -> U/1
  load/1 -> Integrator/1, Fcn/1
  Fcn/1 -> Sum3/2
  U0/1 -> Sum1/1
  Sum1/1 -> Sum3/1
  Integrator/1 -> Scope4/1, Gain/1
  Gain/1 -> Sum1/2

== system Full/Transfer Functions Angles/Винтомоторная группа/CONTROL ROTORS ==
  note: При начальном заряде управляющего аккумулятора
      | 12.6 В начальная тяга 0,6306
      | 11.6 В начальная тяга 0,6001
  Clock1 : Clock
  Sum1 : Sum  Inputs=|++
  Sum2 : Sum  Inputs=|++
  Sum21 : Sum  Inputs=|++
  "Начальное напряжение 1 батареи УД, В" : Constant  Value=11.6
  "Начальное напряжение 2 батареи УД, В" : Constant  Value=11.6
  Снижение тяги при падении напряжения на 1 CR1 : Fcn  Expr=-0.0002809*u(1)
  Снижение тяги при падении напряжения на 1 CR2 : Fcn  Expr=-0.0002809*u(1)
  вычисление начальной тяги 1 CR1 : Fcn  Expr=0.03050*u(1)+0.246299
  вычисление начальной тяги 1 CR2 : Fcn  Expr=0.03050*u(1)+0.246299
  CR Thrust : Outport
  wires:
  Sum21/1 -> Sum2/1
  Sum2/1 -> CR Thrust/1
  "Начальное напряжение 1 батареи УД, В"/1 -> вычисление начальной тяги 1 CR1/1
  Снижение тяги при падении напряжения на 1 CR1/1 -> Sum21/1
  вычисление начальной тяги 1 CR1/1 -> Sum21/2
  Sum1/1 -> Sum2/2
  Clock1/1 -> Снижение тяги при падении напряжения на 1 CR2/1, Снижение тяги при падении напряжения на 1 CR1/1
  "Начальное напряжение 2 батареи УД, В"/1 -> вычисление начальной тяги 1 CR2/1
  Снижение тяги при падении напряжения на 1 CR2/1 -> Sum1/1
  вычисление начальной тяги 1 CR2/1 -> Sum1/2

== system Full/Transfer Functions Angles/Винтомоторная группа/ENGINE ==
  U_in : Inport
  Constant1 : Constant  Value=690
  Constant3 : Constant  Value=0
  Sum1 : Sum  Inputs=|++
  Sum2 : Sum  Inputs=|+-
  Zero_tf4 : TransferFcn  Numerator=[-2112 5.908e04 5061 1.569e04]  Denominator=[1 22.4 155.9 19.71 40.79]
  RPM : Outport
  wires:
  U_in/1 -> Sum2/1
  Zero_tf4/1 -> Sum1/1
  Sum2/1 -> Zero_tf4/1
  Constant1/1 -> Sum1/2
  Constant3/1 -> Sum2/2
  Sum1/1 -> RPM/1

== system Full/Transfer Functions Angles/Винтомоторная группа/ESC ==
  Com : Inport
  U_bat : Inport  Port=2
  Product1 : Product
  U_out : Outport
  wires:
  Product1/1 -> U_out/1
  Com/1 -> Product1/1
  U_bat/1 -> Product1/2

== system Full/Transfer Functions Angles/Винтомоторная группа/MAIN ROTORS ==
  note: P = alpha * ro * n^2 * D^4 + K * n [затенение]
  RPM : Inport
  1st MR1 : Fcn  Expr=5.9e-08*u(1)^2-9.525e-05*u(1)
  Gain : Gain  Gain=2
  MR Thrust : Outport
  wires:
  Gain/1 -> MR Thrust/1
  RPM/1 -> 1st MR1/1
  1st MR1/1 -> Gain/1

== system Full/Динамика/OBJECT/AIR RESISTANCE ==
  note: Индуктивная скорость
  note: -ro/2 * Sfz * (Vz-Vi) * |Vz-Vi|
  note: T/(2*ro*pi*R^2)
  T : Inport
  Vz : Inport  Port=2
  Abs : Abs
  Gain : Gain  Gain=1.29*0.084/2
  Gain1 : Gain  Gain=2
  Gain2 : Gain  Gain=1/(2*1.29*3.1415*0.48^2)
  Gain4 : Gain  Gain=0
  Product1 : Product
  Sqrt : Sqrt  SaturateOnIntegerOverflow=on
  Sum3 : Sum  Inputs=|+-
  V_air : Terminator
  Resistance : Outport
  wires:
  Gain2/1 -> Sqrt/1
  Vz/1 -> Sum3/1
  Abs/1 -> Product1/2
  Product1/1 -> Gain/1
  Gain/1 -> Gain1/1
  Gain1/1 -> Resistance/1
  T/1 -> Gain2/1
  Gain4/1 -> Sum3/2
  Sqrt/1 -> V_air/1, Gain4/1
  Sum3/1 -> Abs/1, Product1/1

== system Full/Динамика/OBJECT/DYNAMICS ==
  T_sum : Inport
  MASS : Inport  Port=2
  Product : Product  Inputs=*/
  Sum1 : Sum  Inputs=|+-
  g1 : Constant  Value=9.81
  Az_dyn : Outport
  Tz : Outport  Port=2
  wires:
  Sum1/1 -> Az_dyn/1
  g1/1 -> Sum1/2
  Product/1 -> Sum1/1
  MASS/1 -> Product/2
  T_sum/1 -> Tz/1, Product/1

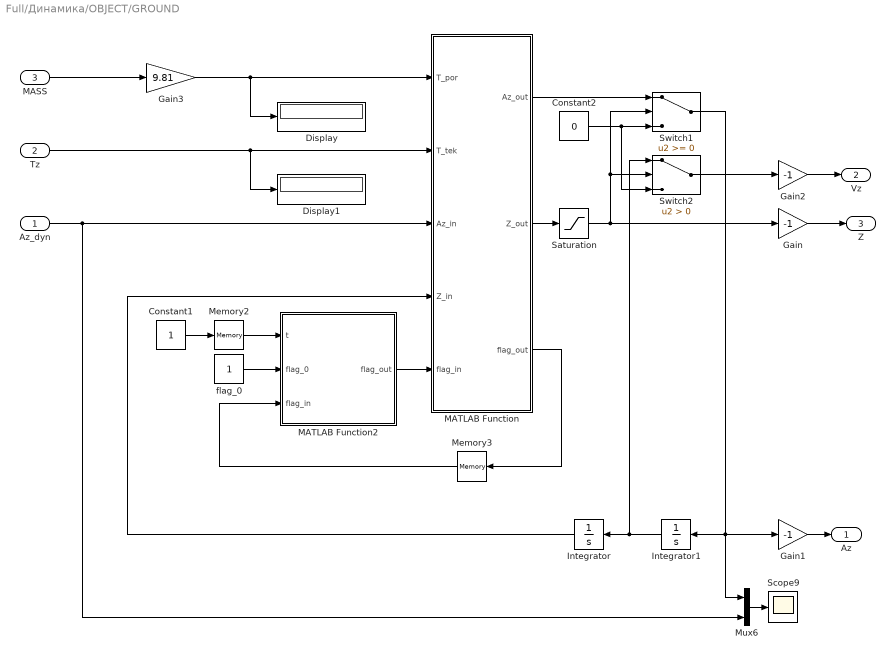
== system Full/Динамика/OBJECT/GROUND ==
  Az_dyn : Inport
  Tz : Inport  Port=2
  MASS : Inport  Port=3
  Constant1 : Constant
  Constant2 : Constant  Value=0
  Display : Display
  Display1 : Display
  Gain : Gain  Gain=-1
  Gain1 : Gain  Gain=-1
  Gain2 : Gain  Gain=-1
  Gain3 : Gain  Gain=9.81
  Integrator : Integrator
  Integrator1 : Integrator
  MATLAB Function : MATLAB Function  TreatAsAtomicUnit=on
  MATLAB Function2 : MATLAB Function  TreatAsAtomicUnit=on
  Memory2 : Memory
  Memory3 : Memory
  Mux6 : Mux  Inputs=2
  Saturation : Saturate  UpperLimit=100  LowerLimit=0
  Scope9 : Scope
      settings: TimeRange=2  YMin=0  YMax=1  SaveName=T_com19
  Switch1 : Switch
  Switch2 : Switch  Criteria=u2 > Threshold
  flag_0 : Constant
  Az : Outport
  Vz : Outport  Port=2
  Z : Outport  Port=3
  wires:
  Saturation/1 -> Switch1/2, Switch2/2, Gain/1
  Switch2/1 -> Gain2/1
  Az_dyn/1 -> Mux6/2, MATLAB Function/3(Az_in)
  Tz/1 -> MATLAB Function/2(T_tek), Display1/1
  MATLAB Function2/1(flag_out) -> MATLAB Function/5(flag_in)
  Memory3/1 -> MATLAB Function2/3(flag_in)
  Memory2/1 -> MATLAB Function2/1(t)
  Constant1/1 -> Memory2/1
  flag_0/1 -> MATLAB Function2/2(flag_0)
  MATLAB Function/3(flag_out) -> Memory3/1
  Integrator1/1 -> Integrator/1, Switch2/1
  Integrator/1 -> MATLAB Function/4(Z_in)
  MASS/1 -> Gain3/1
  MATLAB Function/2(Z_out) -> Saturation/1
  Constant2/1 -> Switch1/3, Switch2/3
  MATLAB Function/1(Az_out) -> Switch1/1
  Gain2/1 -> Vz/1
  Gain/1 -> Z/1
  Switch1/1 -> Mux6/1, Integrator1/1, Gain1/1
  Mux6/1 -> Scope9/1
  Gain1/1 -> Az/1
  Gain3/1 -> MATLAB Function/1(T_por), Display/1

== system Full/Динамика/OBJECT/GROUND EFFECT ==
  note: Отношение высоты
      | плоскости винтов
      | к диаметру
  H_shassi : Inport
  Gain3 : Gain  Gain=-1/0.48
  Gain5 : Gain  Gain=1/100
  Scope1 : Scope
      settings: TimeRange=2  YMin=-0  YMax=2  SaveName=T_com27
  Scope2 : Scope
      settings: TimeRange=2  YMin=0  YMax=1  SaveName=T_com28
  Scope4 : Scope
      settings: TimeRange=2  YMin=110.5  YMax=112  SaveName=T_com24
  Sum28 : Sum  Inputs=|++
  "[0; 1.7]3" : Saturate  UpperLimit=1.7  LowerLimit=0
  "[1; 1.3]" : Saturate  UpperLimit=1.5  LowerLimit=1
  Высота винтов над шасси : Constant  Value=-0.24
  К_gound1 : Fcn  Expr=12.8*u(1)^2-45*u(1)+139.1
  K : Outport
  wires:
  Gain3/1 -> "[0; 1.7]3"/1
  H_shassi/1 -> Scope2/1, Sum28/1
  К_gound1/1 -> Scope4/1, Gain5/1
  "[1; 1.3]"/1 -> Scope1/1, K/1
  Sum28/1 -> Gain3/1
  "[0; 1.7]3"/1 -> К_gound1/1
  Высота винтов над шасси/1 -> Sum28/2
  Gain5/1 -> "[1; 1.3]"/1

== matlab function Full/Disturbance & Aerodynamics/Rotate vind by yaw ==
  data: vx input; loc_VX output; vy input; yaw input; loc_VY output
function [loc_VX,loc_VY] = fcn(vx,vy,yaw)
%#codegen
loc_VX = cos(yaw)*vx + sin(yaw)*vy;
loc_VY = -sin(yaw)*vx + cos(yaw)*vy;

== matlab function Full/Кинематика ==
  data: ATT_Roll input; Fx output; Fy output; ATT_Pitch input; ATT_Yaw input; Thrust input; Fz output; Yaw output
function [Fx,Fy,Fz, Yaw] = fcn(ATT_Roll, ATT_Pitch, ATT_Yaw, Thrust)
%#codegen


Fx =  -sin(ATT_Pitch) * cos(ATT_Yaw) - sin(ATT_Roll) * sin(ATT_Yaw);
Fy =  -sin(ATT_Pitch) * sin(ATT_Yaw) + sin(ATT_Roll) * cos(ATT_Yaw);
Fz = Thrust*cos(ATT_Roll)*cos(ATT_Pitch)*9.81;

Yaw = ATT_Yaw;

== matlab function Full/Динамика/OBJECT/GROUND/MATLAB Function ==
  data: T_por input; T_tek input; Az_out output; Z_out output; Az_in input; Z_in input; flag_out output; flag_in input
function [Az_out, Z_out, flag_out]  = fcn(T_por, T_tek, Az_in, Z_in, flag_in)
%#codegen
flag = flag_in;
Az = 0;
Z = Z_in;

if (T_tek < T_por) && (flag == 0)
    Az = 0;
    Z = 0;
elseif (T_tek >= T_por) && (flag == 0)
    Az = Az_in;
    Z = Z_in;
    flag = 1;
elseif (T_tek >= T_por) && (flag == 1)
    Az = Az_in;
    Z = Z_in;

% elseif (T_tek >= T_por) && (flag == 1) && (Z_in > 0)
%     Az = Az_in;
%     Z = Z_in;
% elseif (T_tek >= T_por) && (flag == 1) && (Z_in <= 0)
%     Az = Az_in;
%     Z = 0;
%     flag = 0;

elseif (T_tek < T_por) && (flag == 1) && (Z_in > 0)
    Az = Az_in;
    Z = Z_in;
elseif (T_tek < T_por) && (flag == 1) && (Z_in <= 0)
    Az = 0;
    Z = 0;
    flag = 0;
end
flag_out = flag;
Az_out = Az;
Z_out = Z;

== matlab function Full/Autopilot_full_30_11_16/XYZ to Angles ==
  data: AX input; RollSP output; AY input; AZ input; LPSP_Yaw input; PitchSP output; YawSP output; ThrustSP output
function [RollSP,PitchSP,YawSP,ThrustSP] = fcn(AX,AY,AZ,LPSP_Yaw)
%#Функция преобразования желаемого вектора поворота в желаемые углы

norm = sqrt(AX*AX + AY*AY + AZ*AZ);
popravka = 1/norm;

RollSP = popravka * (AY * cos(LPSP_Yaw) - AX * sin(LPSP_Yaw));
PitchSP = -popravka * (AY * sin(LPSP_Yaw) + AX * cos(LPSP_Yaw));
ThrustSP = - AZ;
YawSP = LPSP_Yaw;

== matlab function Full/Динамика/OBJECT/GROUND/MATLAB Function2 ==
  data: t input; flag_0 input; flag_in input; flag_out output
function flag_out = fcn(t, flag_0, flag_in)

if t==0
   flag_out = flag_0;
else
   flag_out = flag_in;
end
